simulink model "sampleModel315"  (R2021b)
settings: Solver=VariableStepAuto  StartTime=0.0  StopTime=10.0  RelTol=1e-3
libraries: simulink x3
settings Model: Creator=user  LastModifiedBy=user

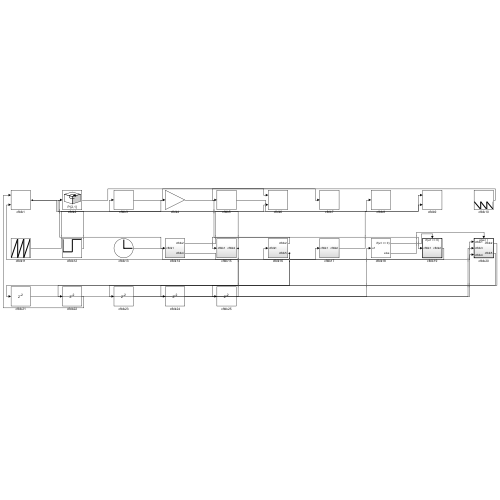
[thumbnail: Simulink's stored preview of the top-level diagram]
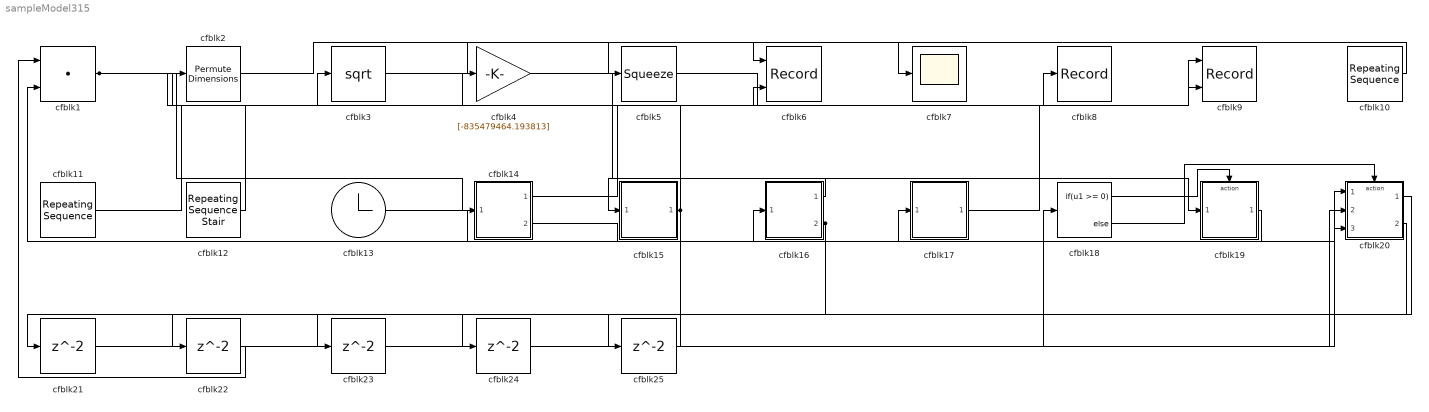
== system sampleModel315 ==
  cfblk1 : DotProduct  InputSameDT=on  OutDataTypeStr=Inherit: Inherit via internal rule
  cfblk10 : simulink/Sources/Repeating Sequence  rep_seq_t=[0 2]  rep_seq_y=[-370065448.541200, -620432923.433621]
  cfblk11 : simulink/Sources/Repeating Sequence  rep_seq_t=[0 2]  rep_seq_y=[-453787971.708335, 158725479.941664]
  cfblk12 : simulink/Sources/Repeating Sequence Stair  OutValues=[187199148.576539, 215844416.780755]  tsamp=-1  OutMin=[]  OutMax=[]  OutDataTypeStr=double  OutputDataTypeScalingMode=double  OutDataType=fixdt(0,8)  ConRadixGroup=Best Precision: Vector-wise  OutScaling=2^-12
  cfblk13 : Clock
  cfblk14 : Subsystem
  cfblk15 : Subsystem
  cfblk16 : Subsystem
  cfblk17 : Subsystem
  cfblk18 : If  IfExpression=u1 >= 0  SampleTime=1
  cfblk19 : Subsystem  TreatAsAtomicUnit=on
  cfblk2 : PermuteDimensions
  cfblk20 : Subsystem  TreatAsAtomicUnit=on
  cfblk{21..25} (5 alike) : Delay  SampleTime=1
  cfblk3 : Sqrt  SaturateOnIntegerOverflow=on
  cfblk4 : Gain  Gain=[-835479464.193813]
  cfblk5 : Squeeze
  cfblk6 : Record  FileSettingsInternal="{\"entries\":[{\"content\":{\"excelSettings\":{\"content\":{},\"type\":\"Streamout.ExcelSettings\"}},\"type\":\"Streamout.FileSettingStorage\",\"uuid\":\"ea7a66c4-707f-43bb-bedd-ce1640931f58\"}],\"packageUris\":[\"http://schema.mathworks.com/mf0/streamout_blocks/R2020a\"],\"version\":\"1.0\"}"  Layout=[1 1]  SignalsInternal="{\"entries\":[{\"content\":{\"signals\":[{\"content\":{\"blockPath\":[\"sampleModel315/cfblk6\"],\"channel\":[],\"dimensions\":[1],\"domain\":\"sampleModel315/cfblk6\",\"lineColor\":\"#a2142f\",\"plots\":[1],\"port\":1,\"sid\":[\"\"],\"signalID\":13337,\"signalName\":\"cfblk3\"},\"type\":\"RecordBlkView.Signal\",\"uuid\":\"fe653821-51d4-4541-9739-7fffe8f9e92c\"},{\"content\":{\"blockPath\":[\"sampleModel315/cfblk6\"],\"channel\":[],\"dimensions\":[1],\"domain\":\"sampleModel315/cfblk6\",\"lineColor\":\"#139fff\",\"plots\":[1],\"port\":2,\"sid\":[\"\"],\"signalID\":13341,\"signalName\":\"cfblk1\"},\"type\":\"RecordBlkView.Signal\",\"uuid\":\"fcec7d04-4f33-4d8f-8f0a-b393c1f90a32\"}]},\"type\":\"RecordBlkView.InputSignals\",\"uuid\":\"3c60eb31-31f2-40ad-9c94-e72c618e0027\"}],\"packageUris\":[\"http://schema.mathworks.com/mf0/streamout_blocks/R2020a\"],\"version\":\"1.0\"}"  VisualizationBindings="{\"xyplotplugin\":{\"info\":[{\"series\":[{\"bindingParametersList\":[{\"parameter\":\"X-Axis\",\"signalID\":13337,\"signalName\":\"cfblk3\"},{\"parameter\":\"Y-Axis\",\"signalID\":13341,\"signalName\":\"cfblk1\"}],\"seriesID\":10539}],\"subplotID\":1}]}}"  CompatibilityTag=XY
  cfblk7 : Scope
  cfblk8 : Record  FileSettingsInternal="{\"entries\":[{\"content\":{\"excelSettings\":{\"content\":{},\"type\":\"Streamout.ExcelSettings\"}},\"type\":\"Streamout.FileSettingStorage\",\"uuid\":\"8bf25dd2-f174-43cd-9488-e6714c33a5c9\"}],\"packageUris\":[\"http://schema.mathworks.com/mf0/streamout_blocks/R2020a\"],\"version\":\"1.0\"}"  SignalsInternal="{\"entries\":[{\"content\":{\"signals\":[{\"content\":{\"blockPath\":[\"sampleModel315/cfblk8\"],\"channel\":[],\"dimensions\":[1],\"domain\":\"sampleModel315/cfblk8\",\"lineColor\":\"#4dbeee\",\"plots\":[1],\"port\":1,\"sid\":[\"\"],\"signalID\":13353,\"signalName\":\"cfblk5\"},\"type\":\"RecordBlkView.Signal\",\"uuid\":\"269b91fc-d16b-480e-b199-f22b9825129f\"}]},\"type\":\"RecordBlkView.InputSignals\",\"uuid\":\"8750209d-f26e-4f01-9684-0c5b6699a606\"}],\"packageUris\":[\"http://schema.mathworks.com/mf0/streamout_blocks/R2020a\"],\"version\":\"1.0\"}"  VisualizationBindings="{\"sparklinesplugin\":{\"info\":[{\"bindingParametersList\":[],\"subplotID\":1}]}}"
  cfblk9 : Record  FileSettingsInternal="{\"entries\":[{\"content\":{\"excelSettings\":{\"content\":{},\"type\":\"Streamout.ExcelSettings\"}},\"type\":\"Streamout.FileSettingStorage\",\"uuid\":\"c631e104-3314-4f0f-b338-028dd409e67b\"}],\"packageUris\":[\"http://schema.mathworks.com/mf0/streamout_blocks/R2020a\"],\"version\":\"1.0\"}"  Layout=[1 1]  SignalsInternal="{\"entries\":[{\"content\":{\"signals\":[{\"content\":{\"blockPath\":[\"sampleModel315/cfblk9\"],\"channel\":[],\"dimensions\":[1],\"domain\":\"sampleModel315/cfblk9\",\"lineColor\":\"#a2142f\",\"plots\":[1],\"port\":1,\"sid\":[\"\"],\"signalID\":13345,\"signalName\":\"cfblk17\"},\"type\":\"RecordBlkView.Signal\",\"uuid\":\"59edc35e-39cc-4277-a006-a3293be3d129\"},{\"content\":{\"blockPath\":[\"sampleModel315/cfblk9\"],\"channel\":[],\"dimensions\":[1],\"domain\":\"sampleModel315/cfblk9\",\"lineColor\":\"#139fff\",\"plots\":[1],\"port\":2,\"sid\":[\"\"],\"signalID\":13349,\"signalName\":\"cfblk14:1\"},\"type\":\"RecordBlkView.Signal\",\"uuid\":\"6a2313a0-5806-4fd2-8022-36b1f11b27b4\"}]},\"type\":\"RecordBlkView.InputSignals\",\"uuid\":\"efe503ed-18a0-43e6-8638-60c0fad12aee\"}],\"packageUris\":[\"http://schema.mathworks.com/mf0/streamout_blocks/R2020a\"],\"version\":\"1.0\"}"  VisualizationBindings="{\"xyplotplugin\":{\"info\":[{\"series\":[{\"bindingParametersList\":[{\"parameter\":\"X-Axis\",\"signalID\":13345,\"signalName\":\"cfblk17\"},{\"parameter\":\"Y-Axis\",\"signalID\":13349,\"signalName\":\"cfblk14:1\"}],\"seriesID\":9879}],\"subplotID\":1}]}}"  CompatibilityTag=XY
  wires:
  cfblk16/1(cfblk2) -> cfblk15/1(cfblk1)
  cfblk13/1 -> cfblk17/1(cfblk1)
  cfblk3/1 -> cfblk6/1
  cfblk15/1(cfblk2) -> cfblk3/1, cfblk21/1
  cfblk1/1 -> cfblk14/1(cfblk1), cfblk6/2
  cfblk19/1(cfblk2) -> cfblk16/1(cfblk1)
  cfblk4/1 -> cfblk19/1(cfblk1)
  cfblk10/1 -> cfblk5/1
  cfblk2/1 -> cfblk7/1
  cfblk12/1 -> cfblk2/1
  cfblk5/1 -> cfblk8/1
  cfblk17/1(cfblk2) -> cfblk9/1
  cfblk11/1 -> cfblk4/1
  cfblk16/2(cfblk5) -> cfblk22/1, cfblk23/1
  cfblk14/1(cfblk2) -> cfblk9/2
  cfblk14/2(cfblk4) -> cfblk20/1(cfblk1)
  cfblk18/1 -> cfblk19/Action
  cfblk18/2 -> cfblk20/Action
  cfblk21/1 -> cfblk20/3(cfblk4)
  cfblk22/1 -> cfblk1/1
  cfblk23/1 -> cfblk20/2(cfblk3)
  cfblk20/1(cfblk2) -> cfblk24/1
  cfblk24/1 -> cfblk18/1
  cfblk20/2(cfblk5) -> cfblk25/1
  cfblk25/1 -> cfblk1/2

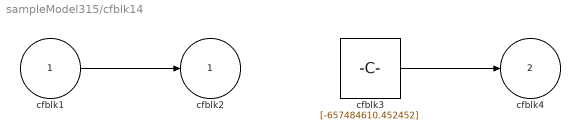
== system sampleModel315/cfblk14 ==
  cfblk1 : Inport
  cfblk3 : Constant  Value=[-657484610.452452]  SampleTime=1
  cfblk2 : Outport
  cfblk4 : Outport  Port=2
  wires:
  cfblk1/1 -> cfblk2/1
  cfblk3/1 -> cfblk4/1

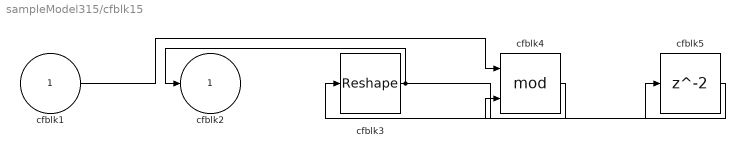
== system sampleModel315/cfblk15 ==
  cfblk1 : Inport
  cfblk3 : Reshape
  cfblk4 : Math  Operator=mod  SaturateOnIntegerOverflow=on
  cfblk5 : Delay  SampleTime=1
  cfblk2 : Outport
  wires:
  cfblk3/1 -> cfblk2/1, cfblk5/1
  cfblk1/1 -> cfblk4/1
  cfblk4/1 -> cfblk3/1
  cfblk5/1 -> cfblk4/2

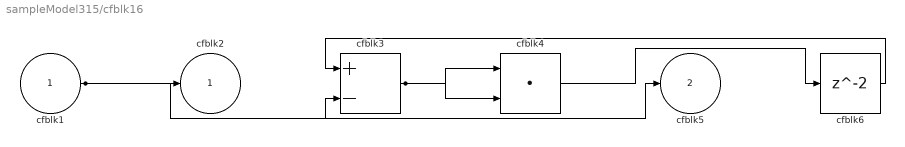
== system sampleModel315/cfblk16 ==
  cfblk1 : Inport
  cfblk3 : Sum  Inputs=+-
  cfblk4 : DotProduct  InputSameDT=on  OutDataTypeStr=Inherit: Inherit via internal rule
  cfblk6 : Delay  SampleTime=1
  cfblk2 : Outport
  cfblk5 : Outport  Port=2
  wires:
  cfblk3/1 -> cfblk4/1, cfblk4/2
  cfblk1/1 -> cfblk5/1, cfblk3/2, cfblk2/1
  cfblk4/1 -> cfblk6/1
  cfblk6/1 -> cfblk3/1

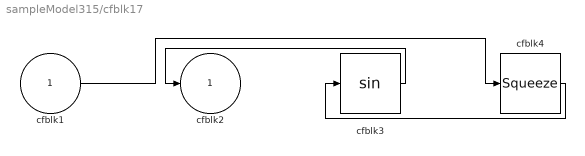
== system sampleModel315/cfblk17 ==
  cfblk1 : Inport
  cfblk3 : Trigonometry
  cfblk4 : Squeeze
  cfblk2 : Outport
  wires:
  cfblk3/1 -> cfblk2/1
  cfblk4/1 -> cfblk3/1
  cfblk1/1 -> cfblk4/1

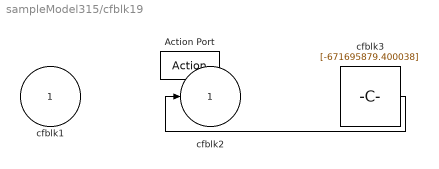
== system sampleModel315/cfblk19 ==
  cfblk1 : Inport
  Action Port : ActionPort  ActionPortLabel=if(u1 >= 0)
  cfblk3 : Constant  Value=[-671695879.400038]  SampleTime=1
  cfblk2 : Outport
  wires:
  cfblk3/1 -> cfblk2/1

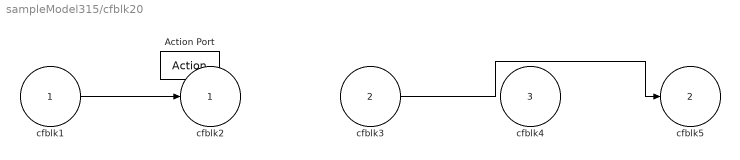
== system sampleModel315/cfblk20 ==
  cfblk1 : Inport
  cfblk3 : Inport  Port=2
  cfblk4 : Inport  Port=3
  Action Port : ActionPort  ActionPortLabel=else
  cfblk2 : Outport
  cfblk5 : Outport  Port=2
  wires:
  cfblk1/1 -> cfblk2/1
  cfblk3/1 -> cfblk5/1
